simulink model "EML_Example"  (R2016a)
settings: Solver=FixedStepAuto  StartTime=0.0  StopTime=10.0  RelTol=1e-3
settings Model: Creator=darenlee  LastModifiedBy=darenlee
settings OptimizationCC: DefaultParameterBehavior=Inlined  OptimizeModelRefInitCode=on  LifeSpan=1
settings SFSimCC: SimCustomHeaderCode="#include \"external_include_file.h\""  SimUserSources=external_src_file.c
settings RTWCC: SystemTargetFile=ert.tlc  TemplateMakefile=ert_default_tmf  GenerateReport=on  IncludeHyperlinkInReport=on  LaunchReport=on  GenerateTraceInfo=on  GenerateTraceReport=on  GenerateTraceReportSl=on  GenerateTraceReportSf=on  GenerateTraceReportEml=on
settings CodeAppCC: ForceParamTrailComments=on  IgnoreCustomStorageClasses=off  OperatorAnnotations=on  SimulinkDataObjDesc=on  SFDataObjDesc=on  MATLABFcnDesc=on  InsertBlockDesc=on  MATLABSourceComments=on
settings ERTTargetCC: GenerateSampleERTMain=on  InlinedParameterPlacement=NonHierarchical  ERTCustomFileTemplate=example_file_process.tlc

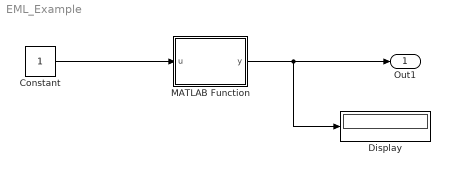
== system EML_Example ==
  Constant : Constant
  Display : Display
  MATLAB Function : MATLAB Function  TreatAsAtomicUnit=on
  Out1 : Outport
  wires:
  Constant/1 -> MATLAB Function/1(u)
  MATLAB Function/1(y) -> Display/1, Out1/1

== matlab function EML_Example/MATLAB Function ==
  data: u input; y output
function y = fcn(u)
%#codegen

if coder.target('rtw') 
    %This is for code generation. Code you write in this if branch will
    %show up in the generated code only
    
    coder.updateBuildInfo('addSourceFiles','external_src_file.c');
    coder.updateBuildInfo('addIncludeFiles','external_include_file.h');
    
    y = 0; %sometimes you need to pre-define your output like this
    coder.ceval('external_function',coder.wref(y),coder.rref(u));
    
else
    %this is for simulation only
    y = u*2;


end



end
